simulink model "Compressor"  (R2023b)
settings: Solver=VariableStepAuto  StartTime=0.0  StopTime=10.0  RelTol=1e-3
undefined symbols (not defined in the file): fs
libraries: ee_lib x38, fl_lib x24, nesl_utility x7
(part 2 of 2)

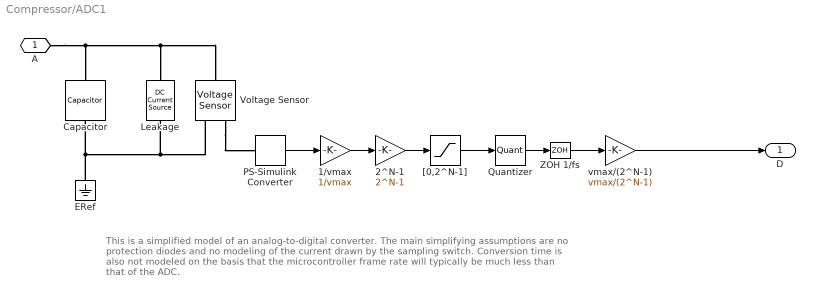
== system Compressor/ADC1 ==
  note: This is a simplified model of an analog-to-digital converter. The main simplifying assumptions
      | are no protection diodes and no modeling of the current drawn by the sampling switch.
      | Conversion time is also not modeled on the basis that the microcontroller frame rate will
      | typically be much less than that of the ADC.
  1/vmax : Gain  Gain=1/vmax
  2^N-1 : Gain  Gain=2^N-1
  Capacitor : fl_lib/Electrical/Electrical Elements/Capacitor  c=1e-6 F  r=1e-6 Ohm  g=0 1/Ohm  i_specify=off  i_priority=High  i=0 A  i_nominal_specify=off  i_nominal_unit=A  i_nominal_value=1  v_specify=off  v_priority=High  v=0 V  v_nominal_specify=off  v_nominal_unit=V  v_nominal_value=1  vc_specify=on  vc_priority=High  vc=0 V  vc_nominal_specify=off  vc_nominal_unit=V  vc_nominal_value=1
  ERef : fl_lib/Electrical/Electrical Elements/Electrical Reference
  Leakage : fl_lib/Electrical/Electrical Sources/DC Current Source  i0=ileak A
      settings: InternalSimscapePortConfiguration="{\"Bottom\":[],\"Left\":[{\"id\":\"p\",\"label\":\"\",\"type\":\"foundation.electrical.electrical\"}],\"Right\":[{\"id\":\"n\",\"label\":\"\",\"type\":\"foundation.electrical.electrical\"}],\"Top\":[]}"
  PS-Simulink Converter : nesl_utility/PS-Simulink Converter  PhysicalDomain=network_engine_domain  SubClassName=ps_output  LeftPortType=input  RightPortType=output  PseudoPeriodic=off  Frequencies=[]  VectorFormat=1-D array  Unit=V  AffineConversion=off
  Quantizer : Quantizer
  Voltage Sensor : fl_lib/Electrical/Electrical Sensors/Voltage Sensor
  ZOH 1/fs : ZeroOrderHold  SampleTime=1/fs
  "[0,2^N-1]" : Saturate  UpperLimit=2^N-1  LowerLimit=0
  vmax/(2^N-1) : Gain  Gain=vmax/(2^N-1)
  A : PMIOPort  Side=Left
  D : Outport  VectorParamsAs1DForOutWhenUnconnected=off
  wires:
  "[0,2^N-1]"/1 -> Quantizer/1
  1/vmax/1 -> 2^N-1/1
  2^N-1/1 -> "[0,2^N-1]"/1
  PS-Simulink Converter/1 -> 1/vmax/1
  ZOH 1/fs/1 -> vmax/(2^N-1)/1
  Quantizer/1 -> ZOH 1/fs/1
  vmax/(2^N-1)/1 -> D/1
  connections:
  A/RConn1 -- Voltage Sensor/LConn1 -- Leakage/RConn1 -- Capacitor/LConn1
  ERef/LConn1 -- Voltage Sensor/RConn2 -- Leakage/LConn1 -- Capacitor/RConn1
  Voltage Sensor/RConn1 -- PS-Simulink Converter/LConn1

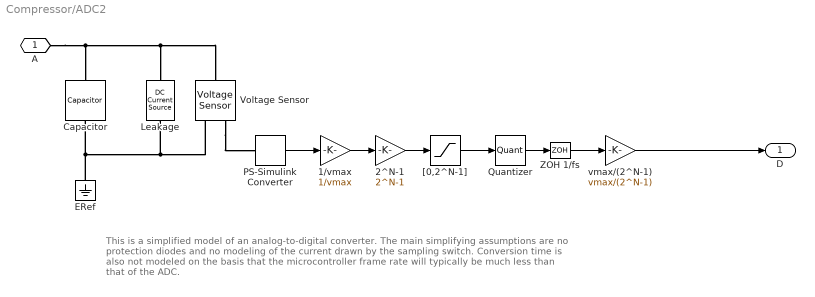
== system Compressor/ADC2 ==
  note: This is a simplified model of an analog-to-digital converter. The main simplifying assumptions
      | are no protection diodes and no modeling of the current drawn by the sampling switch.
      | Conversion time is also not modeled on the basis that the microcontroller frame rate will
      | typically be much less than that of the ADC.
  1/vmax : Gain  Gain=1/vmax
  2^N-1 : Gain  Gain=2^N-1
  Capacitor : fl_lib/Electrical/Electrical Elements/Capacitor  c=1e-6 F  r=1e-6 Ohm  g=0 1/Ohm  i_specify=off  i_priority=High  i=0 A  i_nominal_specify=off  i_nominal_unit=A  i_nominal_value=1  v_specify=off  v_priority=High  v=0 V  v_nominal_specify=off  v_nominal_unit=V  v_nominal_value=1  vc_specify=on  vc_priority=High  vc=0 V  vc_nominal_specify=off  vc_nominal_unit=V  vc_nominal_value=1
  ERef : fl_lib/Electrical/Electrical Elements/Electrical Reference
  Leakage : fl_lib/Electrical/Electrical Sources/DC Current Source  i0=ileak A
      settings: InternalSimscapePortConfiguration="{\"Bottom\":[],\"Left\":[{\"id\":\"p\",\"label\":\"\",\"type\":\"foundation.electrical.electrical\"}],\"Right\":[{\"id\":\"n\",\"label\":\"\",\"type\":\"foundation.electrical.electrical\"}],\"Top\":[]}"
  PS-Simulink Converter : nesl_utility/PS-Simulink Converter  PhysicalDomain=network_engine_domain  SubClassName=ps_output  LeftPortType=input  RightPortType=output  PseudoPeriodic=off  Frequencies=[]  VectorFormat=1-D array  Unit=V  AffineConversion=off
  Quantizer : Quantizer
  Voltage Sensor : fl_lib/Electrical/Electrical Sensors/Voltage Sensor
  ZOH 1/fs : ZeroOrderHold  SampleTime=1/fs
  "[0,2^N-1]" : Saturate  UpperLimit=2^N-1  LowerLimit=0
  vmax/(2^N-1) : Gain  Gain=vmax/(2^N-1)
  A : PMIOPort  Side=Left
  D : Outport  VectorParamsAs1DForOutWhenUnconnected=off
  wires:
  "[0,2^N-1]"/1 -> Quantizer/1
  1/vmax/1 -> 2^N-1/1
  2^N-1/1 -> "[0,2^N-1]"/1
  PS-Simulink Converter/1 -> 1/vmax/1
  ZOH 1/fs/1 -> vmax/(2^N-1)/1
  Quantizer/1 -> ZOH 1/fs/1
  vmax/(2^N-1)/1 -> D/1
  connections:
  A/RConn1 -- Voltage Sensor/LConn1 -- Leakage/RConn1 -- Capacitor/LConn1
  ERef/LConn1 -- Voltage Sensor/RConn2 -- Leakage/LConn1 -- Capacitor/RConn1
  Voltage Sensor/RConn1 -- PS-Simulink Converter/LConn1
